simulink model "divider4bit"  (R2020a)
settings: Solver=VariableStepAuto  StartTime=0.0  StopTime=10.0  RelTol=1e-3
libraries: simulink_extras x4
(part 1 of 2)
settings Model: Creator=kishan  LastModifiedBy=kishan

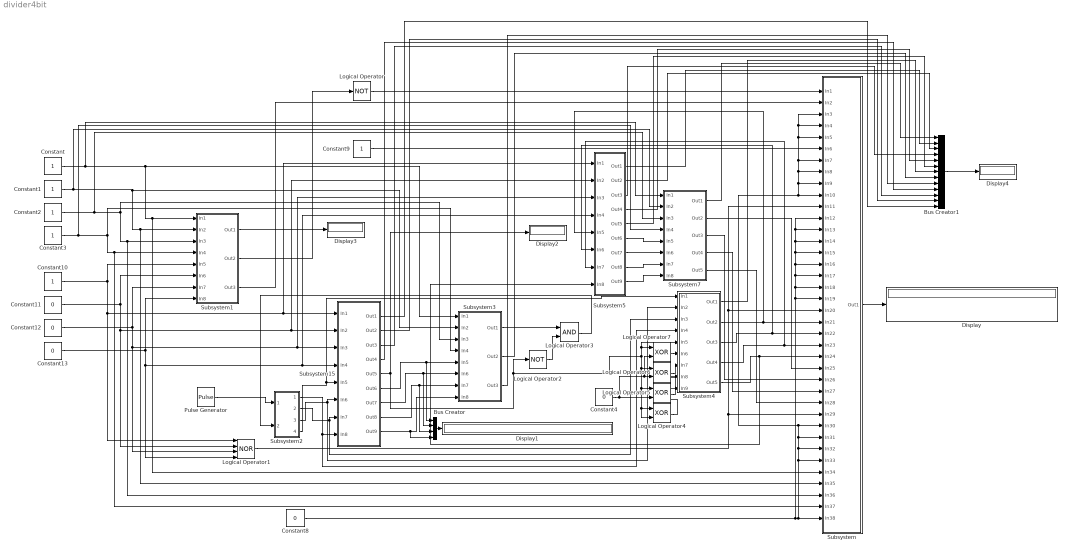
== system divider4bit ==
  Bus Creator : BusCreator  Inputs=4
  Bus Creator1 : BusCreator  Inputs=13
  Constant{,1..3,10} (5 alike) : Constant  OutDataTypeStr=boolean
  Constant11 : Constant  Value=0  OutDataTypeStr=boolean
  Constant12 : Constant  Value=0  OutDataTypeStr=boolean
  Constant13 : Constant  Value=0  OutDataTypeStr=boolean
  Constant4 : Constant  Value=0
  Constant8 : Constant  Value=0
  Constant9 : Constant
  Display{,1..4} (5 alike) : Display
  Logical Operator : Logic  Operator=NOT  AllPortsSameDT=off  OutDataTypeStr=boolean
  Logical Operator1 : Logic  Operator=NOR  Inputs=4  AllPortsSameDT=off  OutDataTypeStr=boolean
  Logical Operator2 : Logic  Operator=NOT  Inputs=4  AllPortsSameDT=off  OutDataTypeStr=boolean
  Logical Operator3 : Logic  AllPortsSameDT=off  OutDataTypeStr=boolean
  Logical Operator{4..7} (4 alike) : Logic  Operator=XOR  AllPortsSameDT=off  OutDataTypeStr=boolean
  Pulse Generator : DiscretePulseGenerator  PulseType=Time based  Period=0.1  PulseWidth=5
  Subsystem : Subsystem
  Subsystem1 : Subsystem
  Subsystem15 : Subsystem
  Subsystem2 : Subsystem
  Subsystem3 : Subsystem
  Subsystem4 : Subsystem
  Subsystem5 : Subsystem
  Subsystem7 : Subsystem
  wires:
  Subsystem/1(Out1) -> Display/1
  Constant3/1 -> Subsystem7/4(In4), Subsystem3/4(In4), Subsystem/37(In37), Subsystem1/4(In4)
  Constant13/1 -> Logical Operator1/4, Subsystem5/4(In4), Subsystem15/4(In4), Subsystem1/8(In8)
  Constant12/1 -> Logical Operator1/3, Subsystem5/3(In3), Subsystem15/3(In3), Subsystem1/7(In7)
  Constant11/1 -> Logical Operator1/2, Subsystem5/2(In2), Subsystem15/2(In2), Subsystem1/6(In6)
  Constant/1 -> Subsystem7/1(In1), Subsystem3/1(In1), Subsystem/34(In34), Subsystem1/1(In1)
  Constant2/1 -> Subsystem7/3(In3), Subsystem3/3(In3), Subsystem/36(In36), Subsystem1/3(In3)
  Subsystem1/3(Out3) -> Subsystem/2(In2)
  Subsystem1/2(Out2) -> Logical Operator/1
  Logical Operator/1 -> Subsystem/1(In1)
  Constant9/1 -> Subsystem/6(In6)
  Logical Operator1/1 -> Subsystem/29(In29), Subsystem/20(In20), Subsystem/11(In11)
  Subsystem15/9(Out9) -> Bus Creator/4, Subsystem3/8(In8)
  Subsystem15/8(Out8) -> Bus Creator/3, Subsystem3/7(In7)
  Subsystem15/7(Out7) -> Bus Creator/2, Subsystem3/6(In6)
  Subsystem15/6(Out6) -> Bus Creator/1, Subsystem3/5(In5)
  Subsystem2/1(Out1) -> Subsystem4/4(In4), Subsystem15/8(In8)
  Subsystem2/2(Out2) -> Subsystem4/3(In3), Subsystem15/7(In7)
  Subsystem2/3(Out3) -> Subsystem4/2(In2), Subsystem15/6(In6)
  Subsystem2/4(Out4) -> Subsystem4/1(In1), Subsystem15/5(In5)
  Pulse Generator/1 -> Subsystem2/1(In1)
  Logical Operator3/1 -> Subsystem2/2(In2)
  Bus Creator/1 -> Display1/1
  Logical Operator2/1 -> Logical Operator3/2
  Subsystem3/1(Out1) -> Logical Operator3/1
  Constant4/1 -> Logical Operator7/2, Logical Operator6/2, Logical Operator5/2
  Logical Operator4/1 -> Subsystem4/9(In9)
  Subsystem4/2(Out2) -> Subsystem5/5(In5), Subsystem/21(In21)
  Subsystem4/3(Out3) -> Subsystem5/6(In6), Subsystem/22(In22)
  Subsystem4/4(Out4) -> Subsystem5/7(In7), Subsystem/23(In23)
  Subsystem4/5(Out5) -> Subsystem/24(In24), Subsystem5/8(In8)
  Subsystem15/5(Out5) -> Logical Operator2/1, Logical Operator5/1, Logical Operator4/2, Logical Operator4/1, Logical Operator6/1, Logical Operator7/1, Subsystem4/5(In5), Display2/1
  Logical Operator5/1 -> Subsystem4/8(In8)
  Logical Operator6/1 -> Subsystem4/7(In7)
  Logical Operator7/1 -> Subsystem4/6(In6)
  Constant10/1 -> Logical Operator1/1, Subsystem5/1(In1), Subsystem15/1(In1), Subsystem1/5(In5)
  Constant1/1 -> Subsystem7/2(In2), Subsystem3/2(In2), Subsystem/35(In35), Subsystem1/2(In2)
  Subsystem5/6(Out6) -> Subsystem7/5(In5)
  Subsystem5/7(Out7) -> Subsystem7/6(In6)
  Subsystem5/8(Out8) -> Subsystem7/7(In7)
  Subsystem5/9(Out9) -> Subsystem7/8(In8)
  Subsystem7/2(Out2) -> Subsystem/25(In25)
  Subsystem7/3(Out3) -> Subsystem/26(In26)
  Subsystem7/4(Out4) -> Subsystem/27(In27)
  Subsystem7/5(Out5) -> Subsystem/28(In28)
  Subsystem1/1(Out1) -> Display3/1
  Constant8/1 -> Subsystem/19(In19), Subsystem/18(In18), Subsystem/17(In17), Subsystem/16(In16), Subsystem/15(In15), Subsystem/14(In14), Subsystem/13(In13), Subsystem/12(In12), Subsystem/38(In38), Subsystem/32(In32), Subsystem/10(In10), Subsystem/9(In9), Subsystem/8(In8), Subsystem/7(In7), Subsystem/5(In5), Subsystem/4(In4), Subsystem/3(In3), Subsystem/30(In30), Subsystem/31(In31), Subsystem/33(In33)
  Bus Creator1/1 -> Display4/1
  Subsystem7/1(Out1) -> Bus Creator1/1
  Subsystem5/1(Out1) -> Bus Creator1/2
  Subsystem5/2(Out2) -> Bus Creator1/3
  Subsystem5/3(Out3) -> Bus Creator1/4
  Subsystem5/4(Out4) -> Bus Creator1/5
  Subsystem5/5(Out5) -> Bus Creator1/6
  Subsystem4/1(Out1) -> Bus Creator1/7
  Subsystem3/2(Out2) -> Bus Creator1/8
  Subsystem3/3(Out3) -> Bus Creator1/9
  Subsystem15/4(Out4) -> Bus Creator1/10
  Subsystem15/3(Out3) -> Bus Creator1/11
  Subsystem15/2(Out2) -> Bus Creator1/12
  Subsystem15/1(Out1) -> Bus Creator1/13

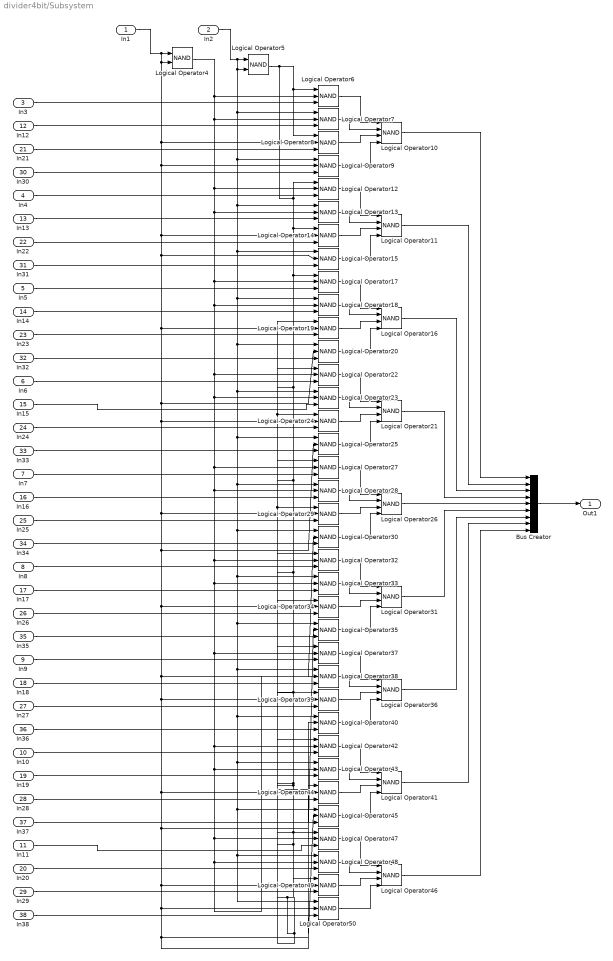
== system divider4bit/Subsystem ==
  In1 : Inport
  In2 : Inport  Port=2
  In3 : Inport  Port=3
  In4 : Inport  Port=4
  In5 : Inport  Port=5
  In6 : Inport  Port=6
  In7 : Inport  Port=7
  In8 : Inport  Port=8
  In9 : Inport  Port=9
  In10 : Inport  Port=10
  In11 : Inport  Port=11
  In12 : Inport  Port=12
  In13 : Inport  Port=13
  In14 : Inport  Port=14
  In15 : Inport  Port=15
  In16 : Inport  Port=16
  In17 : Inport  Port=17
  In18 : Inport  Port=18
  In19 : Inport  Port=19
  In20 : Inport  Port=20
  In21 : Inport  Port=21
  In22 : Inport  Port=22
  In23 : Inport  Port=23
  In24 : Inport  Port=24
  In25 : Inport  Port=25
  In26 : Inport  Port=26
  In27 : Inport  Port=27
  In28 : Inport  Port=28
  In29 : Inport  Port=29
  In30 : Inport  Port=30
  In31 : Inport  Port=31
  In32 : Inport  Port=32
  In33 : Inport  Port=33
  In34 : Inport  Port=34
  In35 : Inport  Port=35
  In36 : Inport  Port=36
  In37 : Inport  Port=37
  In38 : Inport  Port=38
  Bus Creator : BusCreator  Inputs=9
  Logical Operator{10..11,16,21,26,31,36,41,46} (9 alike) : Logic  Operator=NAND  Inputs=4  AllPortsSameDT=off  OutDataTypeStr=boolean
  Logical Operator{6..9,12..15,17..20,22..25,27..30,32..35,37..40,42..45,47..50} (36 alike) : Logic  Operator=NAND  Inputs=3  AllPortsSameDT=off  OutDataTypeStr=boolean
  Logical Operator4 : Logic  Operator=NAND  AllPortsSameDT=off  OutDataTypeStr=boolean
  Logical Operator5 : Logic  Operator=NAND  AllPortsSameDT=off  OutDataTypeStr=boolean
  Out1 : Outport
  wires:
  Logical Operator28/1 -> Logical Operator26/2
  Logical Operator49/1 -> Logical Operator46/3
  In15/1 -> Logical Operator23/3
  In30/1 -> Logical Operator9/3
  Logical Operator33/1 -> Logical Operator31/2
  Logical Operator32/1 -> Logical Operator31/1
  Logical Operator43/1 -> Logical Operator41/2
  Logical Operator37/1 -> Logical Operator36/1
  Logical Operator24/1 -> Logical Operator21/3
  In33/1 -> Logical Operator25/3
  Logical Operator45/1 -> Logical Operator41/4
  Logical Operator42/1 -> Logical Operator41/1
  In37/1 -> Logical Operator45/3
  Logical Operator44/1 -> Logical Operator41/3
  Logical Operator30/1 -> Logical Operator26/4
  In19/1 -> Logical Operator43/3
  In28/1 -> Logical Operator44/3
  Logical Operator34/1 -> Logical Operator31/3
  In38/1 -> Logical Operator50/3
  Logical Operator11/1 -> Bus Creator/2
  Logical Operator22/1 -> Logical Operator21/1
  In18/1 -> Logical Operator38/3
  In22/1 -> Logical Operator14/3
  In14/1 -> Logical Operator18/3
  Logical Operator19/1 -> Logical Operator16/3
  In32/1 -> Logical Operator20/3
  Logical Operator20/1 -> Logical Operator16/4
  Logical Operator48/1 -> Logical Operator46/2
  Logical Operator13/1 -> Logical Operator11/2
  Logical Operator25/1 -> Logical Operator21/4
  In24/1 -> Logical Operator24/3
  In25/1 -> Logical Operator29/3
  In7/1 -> Logical Operator27/3
  In21/1 -> Logical Operator8/3
  Logical Operator23/1 -> Logical Operator21/2
  In8/1 -> Logical Operator32/3
  Logical Operator17/1 -> Logical Operator16/1
  In29/1 -> Logical Operator49/3
  Logical Operator36/1 -> Bus Creator/7
  Logical Operator16/1 -> Bus Creator/3
  In26/1 -> Logical Operator34/3
  Logical Operator50/1 -> Logical Operator46/4
  In17/1 -> Logical Operator33/3
  In3/1 -> Logical Operator6/3
  In4/1 -> Logical Operator12/3
  Logical Operator14/1 -> Logical Operator11/3
  Logical Operator46/1 -> Bus Creator/9
  Logical Operator9/1 -> Logical Operator10/4
  In5/1 -> Logical Operator17/3
  Bus Creator/1 -> Out1/1
  Logical Operator35/1 -> Logical Operator31/4
  Logical Operator26/1 -> Bus Creator/5
  Logical Operator10/1 -> Bus Creator/1
  Logical Operator40/1 -> Logical Operator36/4
  In36/1 -> Logical Operator40/3
  Logical Operator39/1 -> Logical Operator36/3
  In35/1 -> Logical Operator35/3
  Logical Operator29/1 -> Logical Operator26/3
  In2/1 -> Logical Operator50/1, Logical Operator48/1, Logical Operator45/1, Logical Operator43/1, Logical Operator40/1, Logical Operator38/1, Logical Operator35/1, Logical Operator33/1, Logical Operator30/1, Logical Operator28/1, Logical Operator25/1, Logical Operator23/1, Logical Operator20/1, Logical Operator18/1, Logical Operator15/1, Logical Operator13/1, Logical Operator9/1, Logical Operator7/1, Logical Operator5/2, Logical Operator5/1
  Logical Operator38/1 -> Logical Operator36/2
  Logical Operator18/1 -> Logical Operator16/2
  Logical Operator15/1 -> Logical Operator11/4
  In16/1 -> Logical Operator28/3
  Logical Operator27/1 -> Logical Operator26/1
  In27/1 -> Logical Operator39/3
  In20/1 -> Logical Operator48/3
  In10/1 -> Logical Operator42/3
  Logical Operator47/1 -> Logical Operator46/1
  Logical Operator31/1 -> Bus Creator/6
  Logical Operator41/1 -> Bus Creator/8
  In31/1 -> Logical Operator15/3
  Logical Operator8/1 -> Logical Operator10/3
  Logical Operator6/1 -> Logical Operator10/1
  In34/1 -> Logical Operator30/3
  Logical Operator12/1 -> Logical Operator11/1
  In11/1 -> Logical Operator47/3
  In13/1 -> Logical Operator13/3
  Logical Operator7/1 -> Logical Operator10/2
  In12/1 -> Logical Operator7/3
  In23/1 -> Logical Operator19/3
  Logical Operator4/1 -> Logical Operator38/2, Logical Operator48/2, Logical Operator47/2, Logical Operator43/2, Logical Operator42/2, Logical Operator37/2, Logical Operator33/2, Logical Operator32/2, Logical Operator28/2, Logical Operator27/2, Logical Operator23/2, Logical Operator22/2, Logical Operator18/2, Logical Operator17/2, Logical Operator13/2, Logical Operator12/2, Logical Operator7/2, Logical Operator6/2
  Logical Operator21/1 -> Bus Creator/4
  Logical Operator5/1 -> Logical Operator22/1, Logical Operator24/1, Logical Operator29/1, Logical Operator27/1, Logical Operator47/1, Logical Operator49/1, Logical Operator44/1, Logical Operator42/1, Logical Operator37/1, Logical Operator39/1, Logical Operator34/1, Logical Operator32/1, Logical Operator19/1, Logical Operator17/1, Logical Operator14/1, Logical Operator12/1, Logical Operator8/1, Logical Operator6/1
  In9/1 -> Logical Operator37/3
  In1/1 -> Logical Operator40/2, Logical Operator45/2, Logical Operator50/2, Logical Operator49/2, Logical Operator35/2, Logical Operator44/2, Logical Operator39/2, Logical Operator30/2, Logical Operator34/2, Logical Operator25/2, Logical Operator29/2, Logical Operator24/2, Logical Operator20/2, Logical Operator19/2, Logical Operator15/2, Logical Operator14/2, Logical Operator9/2, Logical Operator8/2, Logical Operator4/2, Logical Operator4/1
  In6/1 -> Logical Operator22/3

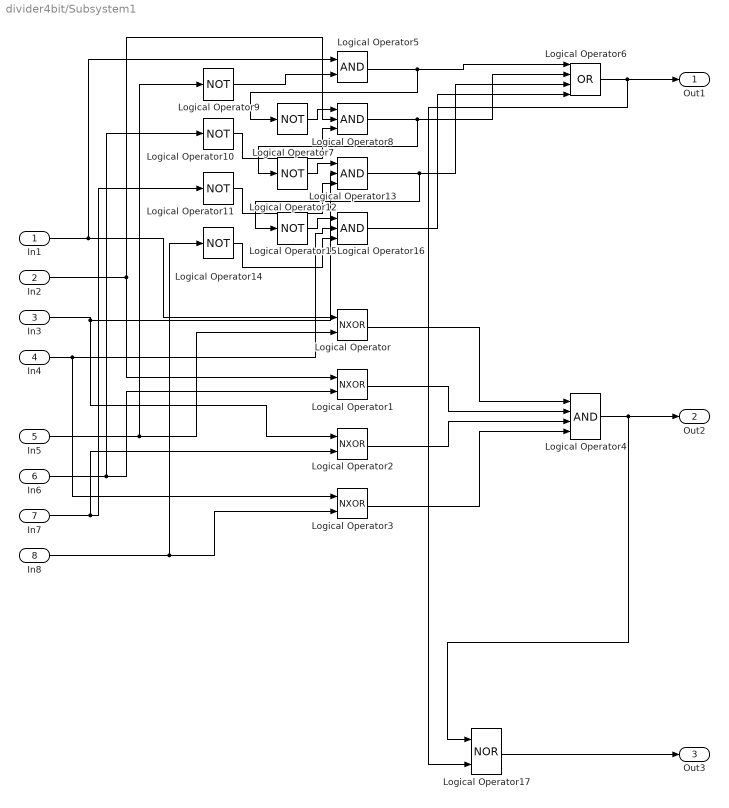
== system divider4bit/Subsystem1 ==
  In1 : Inport
  In2 : Inport  Port=2
  In3 : Inport  Port=3
  In4 : Inport  Port=4
  In5 : Inport  Port=5
  In6 : Inport  Port=6
  In7 : Inport  Port=7
  In8 : Inport  Port=8
  Logical Operator{,1..3} (4 alike) : Logic  Operator=NXOR  AllPortsSameDT=off  OutDataTypeStr=boolean
  Logical Operator{7,9..12,14..15} (7 alike) : Logic  Operator=NOT  Inputs=3  AllPortsSameDT=off  OutDataTypeStr=boolean
  Logical Operator13 : Logic  Inputs=3  AllPortsSameDT=off  OutDataTypeStr=boolean
  Logical Operator16 : Logic  Inputs=3  AllPortsSameDT=off  OutDataTypeStr=boolean
  Logical Operator17 : Logic  Operator=NOR  AllPortsSameDT=off  OutDataTypeStr=boolean
  Logical Operator4 : Logic  Inputs=4  AllPortsSameDT=off  OutDataTypeStr=boolean
  Logical Operator5 : Logic  AllPortsSameDT=off  OutDataTypeStr=boolean
  Logical Operator6 : Logic  Operator=OR  Inputs=4  AllPortsSameDT=off  OutDataTypeStr=boolean
  Logical Operator8 : Logic  Inputs=3  AllPortsSameDT=off  OutDataTypeStr=boolean
  Out1 : Outport
  Out2 : Outport  Port=2
  Out3 : Outport  Port=3
  wires:
  Logical Operator7/1 -> Logical Operator8/1
  Logical Operator17/1 -> Out3/1
  Logical Operator16/1 -> Logical Operator6/4
  Logical Operator12/1 -> Logical Operator13/1
  In7/1 -> Logical Operator11/1, Logical Operator2/2
  Logical Operator4/1 -> Out2/1, Logical Operator17/1
  In1/1 -> Logical Operator5/1, Logical Operator/1
  Logical Operator3/1 -> Logical Operator4/4
  Logical Operator5/1 -> Logical Operator7/1, Logical Operator6/1
  Logical Operator6/1 -> Out1/1, Logical Operator17/2
  In5/1 -> Logical Operator9/1, Logical Operator/2
  In3/1 -> Logical Operator13/2, Logical Operator2/1
  Logical Operator/1 -> Logical Operator4/1
  In6/1 -> Logical Operator10/1, Logical Operator1/2
  Logical Operator1/1 -> Logical Operator4/2
  In4/1 -> Logical Operator16/2, Logical Operator3/1
  In2/1 -> Logical Operator8/2, Logical Operator1/1
  Logical Operator15/1 -> Logical Operator16/1
  In8/1 -> Logical Operator14/1, Logical Operator3/2
  Logical Operator13/1 -> Logical Operator15/1, Logical Operator6/3
  Logical Operator11/1 -> Logical Operator13/3
  Logical Operator8/1 -> Logical Operator12/1, Logical Operator6/2
  Logical Operator2/1 -> Logical Operator4/3
  Logical Operator9/1 -> Logical Operator5/2
  Logical Operator14/1 -> Logical Operator16/3
  Logical Operator10/1 -> Logical Operator8/3

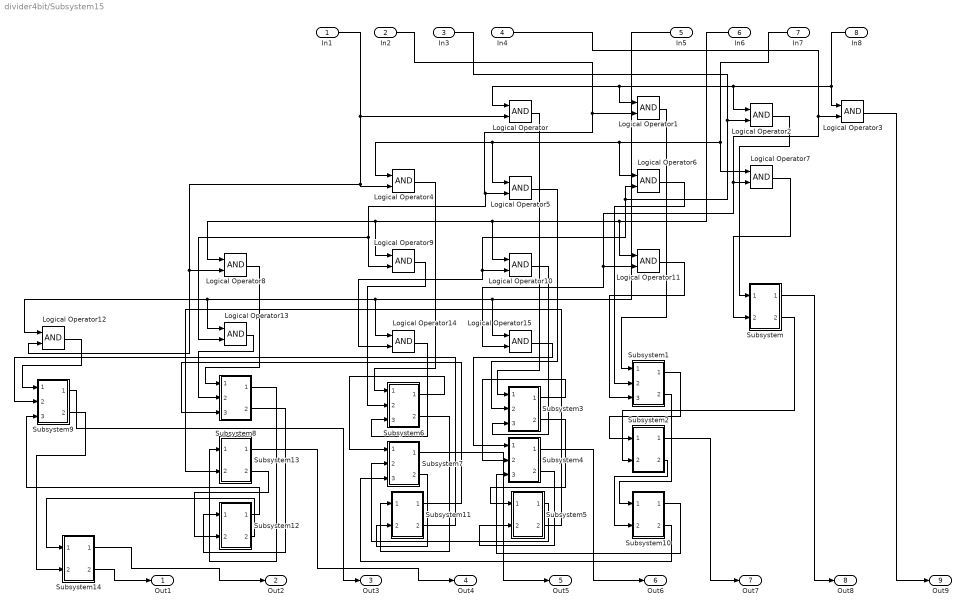
== system divider4bit/Subsystem15 ==
  In1 : Inport
  In2 : Inport  Port=2
  In3 : Inport  Port=3
  In4 : Inport  Port=4
  In5 : Inport  Port=5
  In6 : Inport  Port=6
  In7 : Inport  Port=7
  In8 : Inport  Port=8
  Logical Operator{,1..15} (16 alike) : Logic  AllPortsSameDT=off  OutDataTypeStr=boolean
  Subsystem : Subsystem
  Subsystem1 : Subsystem
  Subsystem10 : Subsystem
  Subsystem11 : Subsystem
  Subsystem12 : Subsystem
  Subsystem13 : Subsystem
  Subsystem14 : Subsystem
  Subsystem2 : Subsystem
  Subsystem3 : Subsystem
  Subsystem4 : Subsystem
  Subsystem5 : Subsystem
  Subsystem6 : Subsystem
  Subsystem7 : Subsystem
  Subsystem8 : Subsystem
  Subsystem9 : Subsystem
  Out1 : Outport
  Out2 : Outport  Port=2
  Out3 : Outport  Port=3
  Out4 : Outport  Port=4
  Out5 : Outport  Port=5
  Out6 : Outport  Port=6
  Out7 : Outport  Port=7
  Out8 : Outport  Port=8
  Out9 : Outport  Port=9
  wires:
  Subsystem11/2(Out2) -> Subsystem9/2(In2)
  Logical Operator7/1 -> Subsystem/2(In2)
  Subsystem4/2(Out2) -> Subsystem5/2(In2)
  Logical Operator13/1 -> Subsystem8/2(In2)
  Subsystem12/1(Out1) -> Subsystem9/3(In3)
  Logical Operator/1 -> Subsystem3/1(In1)
  Subsystem3/1(Out1) -> Subsystem4/2(In2)
  Subsystem14/1(Out1) -> Out2/1
  Logical Operator4/1 -> Subsystem6/1(In1)
  Subsystem1/2(Out2) -> Subsystem10/1(In1)
  Subsystem5/1(Out1) -> Subsystem7/2(In2)
  Subsystem10/2(Out2) -> Subsystem7/3(In3)
  In3/1 -> Logical Operator6/2, Logical Operator14/2, Logical Operator10/2, Logical Operator2/2
  Subsystem8/2(Out2) -> Subsystem12/1(In1)
  Subsystem4/1(Out1) -> Out6/1
  Logical Operator6/1 -> Subsystem1/2(In2)
  Subsystem13/1(Out1) -> Out4/1
  Subsystem2/1(Out1) -> Out7/1
  Subsystem/1(Out1) -> Out8/1
  In5/1 -> Logical Operator12/1, Logical Operator13/1, Logical Operator14/1, Logical Operator15/1
  In1/1 -> Logical Operator12/2, Logical Operator8/2, Logical Operator4/2, Logical Operator/2
  Logical Operator2/1 -> Subsystem/1(In1)
  Subsystem/2(Out2) -> Subsystem2/2(In2)
  Logical Operator3/1 -> Out9/1
  In2/1 -> Logical Operator9/2, Logical Operator13/2, Logical Operator5/2, Logical Operator1/2
  In6/1 -> Logical Operator8/1, Logical Operator9/1, Logical Operator10/1, Logical Operator11/1
  In8/1 -> Logical Operator/1, Logical Operator1/1, Logical Operator2/1, Logical Operator3/1
  Subsystem13/2(Out2) -> Subsystem12/2(In2)
  Logical Operator1/1 -> Subsystem1/1(In1)
  In7/1 -> Logical Operator4/1, Logical Operator5/1, Logical Operator6/1, Logical Operator7/1
  Logical Operator11/1 -> Subsystem1/3(In3)
  Subsystem12/2(Out2) -> Subsystem14/1(In1)
  Logical Operator12/1 -> Subsystem9/1(In1)
  Subsystem10/1(Out1) -> Subsystem4/3(In3)
  Logical Operator15/1 -> Subsystem4/1(In1)
  Logical Operator5/1 -> Subsystem3/2(In2)
  Subsystem7/1(Out1) -> Out5/1
  Subsystem6/2(Out2) -> Subsystem11/1(In1)
  Logical Operator8/1 -> Subsystem8/1(In1)
  Subsystem3/2(Out2) -> Subsystem5/1(In1)
  In4/1 -> Logical Operator15/2, Logical Operator11/2, Logical Operator7/2, Logical Operator3/2
  Subsystem9/1(Out1) -> Out3/1
  Logical Operator14/1 -> Subsystem6/3(In3)
  Subsystem9/2(Out2) -> Subsystem14/2(In2)
  Subsystem11/1(Out1) -> Subsystem8/3(In3)
  Subsystem8/1(Out1) -> Subsystem13/1(In1)
  Subsystem1/1(Out1) -> Subsystem2/1(In1)
  Subsystem2/2(Out2) -> Subsystem10/2(In2)
  Subsystem6/1(Out1) -> Subsystem7/1(In1)
  Subsystem5/2(Out2) -> Subsystem13/2(In2)
  Subsystem14/2(Out2) -> Out1/1
  Logical Operator10/1 -> Subsystem3/3(In3)
  Logical Operator9/1 -> Subsystem6/2(In2)
  Subsystem7/2(Out2) -> Subsystem11/2(In2)

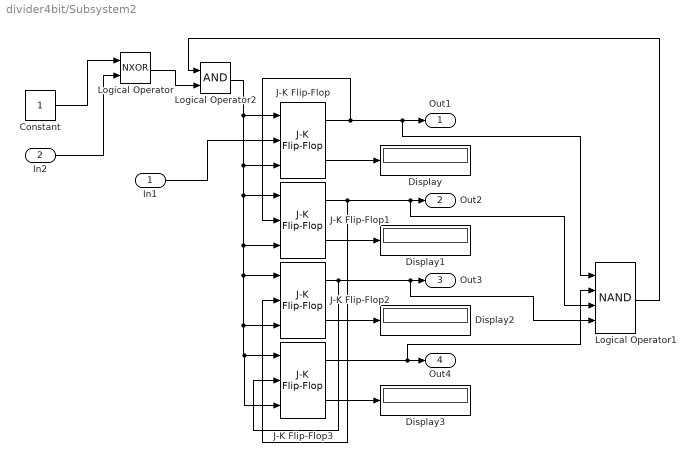
== system divider4bit/Subsystem2 ==
  In1 : Inport
  In2 : Inport  Port=2
  Constant : Constant  OutDataTypeStr=boolean
  Display{,1..3} (4 alike) : Display
  J-K Flip-Flop{,1..3} (4 alike) : simulink_extras/Flip Flops/J-K Flip-Flop  initial_condition=0
  Logical Operator : Logic  Operator=NXOR  AllPortsSameDT=off  OutDataTypeStr=boolean
  Logical Operator1 : Logic  Operator=NAND  Inputs=4  AllPortsSameDT=off  OutDataTypeStr=boolean
  Logical Operator2 : Logic  AllPortsSameDT=off  OutDataTypeStr=boolean
  Out1 : Outport
  Out2 : Outport  Port=2
  Out3 : Outport  Port=3
  Out4 : Outport  Port=4
  wires:
  J-K Flip-Flop1/2 -> Display1/1
  J-K Flip-Flop3/2 -> Display3/1
  J-K Flip-Flop2/2 -> Display2/1
  J-K Flip-Flop3/1 -> Logical Operator1/2, Out4/1
  J-K Flip-Flop/2 -> Display/1
  J-K Flip-Flop1/1 -> J-K Flip-Flop2/2, Logical Operator1/3, Out2/1
  J-K Flip-Flop2/1 -> J-K Flip-Flop3/2, Logical Operator1/4, Out3/1
  In1/1 -> J-K Flip-Flop/2
  J-K Flip-Flop/1 -> J-K Flip-Flop1/2, Logical Operator1/1, Out1/1
  Logical Operator2/1 -> J-K Flip-Flop3/3, J-K Flip-Flop3/1, J-K Flip-Flop2/3, J-K Flip-Flop2/1, J-K Flip-Flop1/3, J-K Flip-Flop1/1, J-K Flip-Flop/3, J-K Flip-Flop/1
  Constant/1 -> Logical Operator/1
  In2/1 -> Logical Operator/2
  Logical Operator/1 -> Logical Operator2/2
  Logical Operator1/1 -> Logical Operator2/1

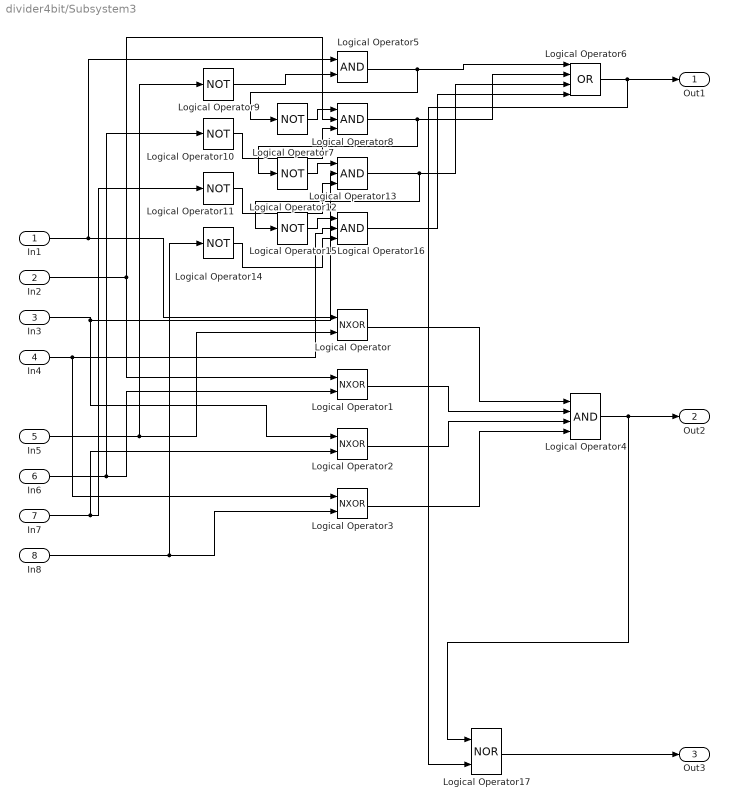
== system divider4bit/Subsystem3 ==
  In1 : Inport
  In2 : Inport  Port=2
  In3 : Inport  Port=3
  In4 : Inport  Port=4
  In5 : Inport  Port=5
  In6 : Inport  Port=6
  In7 : Inport  Port=7
  In8 : Inport  Port=8
  Logical Operator{,1..3} (4 alike) : Logic  Operator=NXOR  AllPortsSameDT=off  OutDataTypeStr=boolean
  Logical Operator{7,9..12,14..15} (7 alike) : Logic  Operator=NOT  Inputs=3  AllPortsSameDT=off  OutDataTypeStr=boolean
  Logical Operator13 : Logic  Inputs=3  AllPortsSameDT=off  OutDataTypeStr=boolean
  Logical Operator16 : Logic  Inputs=3  AllPortsSameDT=off  OutDataTypeStr=boolean
  Logical Operator17 : Logic  Operator=NOR  AllPortsSameDT=off  OutDataTypeStr=boolean
  Logical Operator4 : Logic  Inputs=4  AllPortsSameDT=off  OutDataTypeStr=boolean
  Logical Operator5 : Logic  AllPortsSameDT=off  OutDataTypeStr=boolean
  Logical Operator6 : Logic  Operator=OR  Inputs=4  AllPortsSameDT=off  OutDataTypeStr=boolean
  Logical Operator8 : Logic  Inputs=3  AllPortsSameDT=off  OutDataTypeStr=boolean
  Out1 : Outport
  Out2 : Outport  Port=2
  Out3 : Outport  Port=3
  wires:
  Logical Operator7/1 -> Logical Operator8/1
  Logical Operator17/1 -> Out3/1
  Logical Operator16/1 -> Logical Operator6/4
  Logical Operator12/1 -> Logical Operator13/1
  In7/1 -> Logical Operator11/1, Logical Operator2/2
  Logical Operator4/1 -> Out2/1, Logical Operator17/1
  In1/1 -> Logical Operator5/1, Logical Operator/1
  Logical Operator3/1 -> Logical Operator4/4
  Logical Operator5/1 -> Logical Operator7/1, Logical Operator6/1
  Logical Operator6/1 -> Out1/1, Logical Operator17/2
  In5/1 -> Logical Operator9/1, Logical Operator/2
  In3/1 -> Logical Operator13/2, Logical Operator2/1
  Logical Operator/1 -> Logical Operator4/1
  In6/1 -> Logical Operator10/1, Logical Operator1/2
  Logical Operator1/1 -> Logical Operator4/2
  In4/1 -> Logical Operator16/2, Logical Operator3/1
  In2/1 -> Logical Operator8/2, Logical Operator1/1
  Logical Operator15/1 -> Logical Operator16/1
  In8/1 -> Logical Operator14/1, Logical Operator3/2
  Logical Operator13/1 -> Logical Operator15/1, Logical Operator6/3
  Logical Operator11/1 -> Logical Operator13/3
  Logical Operator8/1 -> Logical Operator12/1, Logical Operator6/2
  Logical Operator2/1 -> Logical Operator4/3
  Logical Operator9/1 -> Logical Operator5/2
  Logical Operator14/1 -> Logical Operator16/3
  Logical Operator10/1 -> Logical Operator8/3

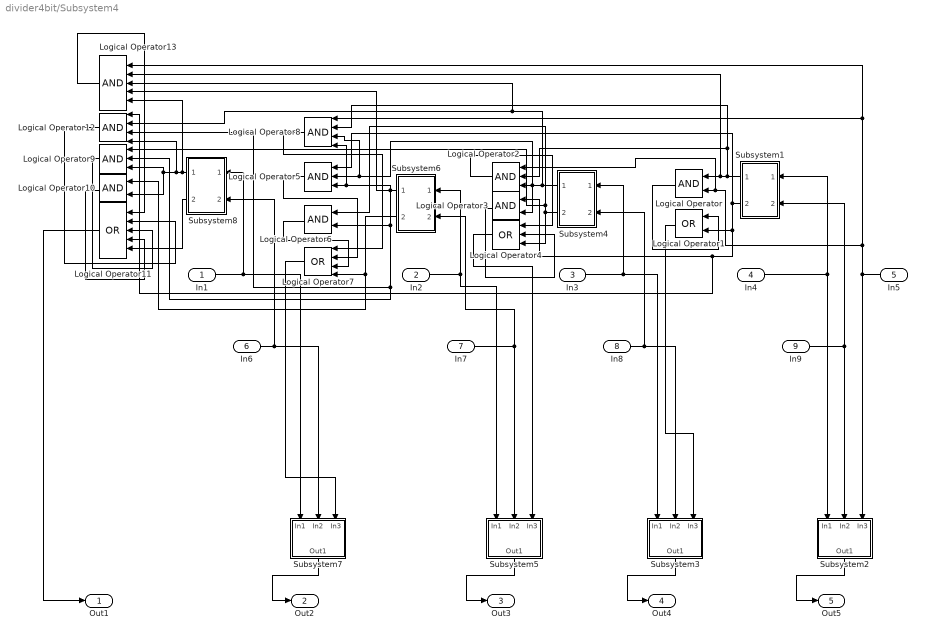
== system divider4bit/Subsystem4 ==
  In1 : Inport
  In2 : Inport  Port=2
  In3 : Inport  Port=3
  In4 : Inport  Port=4
  In5 : Inport  Port=5
  In6 : Inport  Port=6
  In7 : Inport  Port=7
  In8 : Inport  Port=8
  In9 : Inport  Port=9
  Logical Operator{,3,6,10} (4 alike) : Logic  AllPortsSameDT=off  OutDataTypeStr=boolean
  Logical Operator1 : Logic  Operator=OR  AllPortsSameDT=off  OutDataTypeStr=boolean
  Logical Operator11 : Logic  Operator=OR  Inputs=5  AllPortsSameDT=off  OutDataTypeStr=boolean
  Logical Operator12 : Logic  Inputs=4  AllPortsSameDT=off  OutDataTypeStr=boolean
  Logical Operator13 : Logic  Inputs=5  AllPortsSameDT=off  OutDataTypeStr=boolean
  Logical Operator2 : Logic  Inputs=3  AllPortsSameDT=off  OutDataTypeStr=boolean
  Logical Operator4 : Logic  Operator=OR  Inputs=3  AllPortsSameDT=off  OutDataTypeStr=boolean
  Logical Operator5 : Logic  Inputs=3  AllPortsSameDT=off  OutDataTypeStr=boolean
  Logical Operator7 : Logic  Operator=OR  Inputs=4  AllPortsSameDT=off  OutDataTypeStr=boolean
  Logical Operator8 : Logic  Inputs=4  AllPortsSameDT=off  OutDataTypeStr=boolean
  Logical Operator9 : Logic  Inputs=3  AllPortsSameDT=off  OutDataTypeStr=boolean
  Subsystem1 : Subsystem
  Subsystem2 : Subsystem
  Subsystem3 : Subsystem
  Subsystem4 : Subsystem
  Subsystem5 : Subsystem
  Subsystem6 : Subsystem
  Subsystem7 : Subsystem
  Subsystem8 : Subsystem
  Out1 : Outport
  Out2 : Outport  Port=2
  Out3 : Outport  Port=3
  Out4 : Outport  Port=4
  Out5 : Outport  Port=5
  wires:
  Logical Operator11/1 -> Out1/1
  Logical Operator5/1 -> Logical Operator7/2
  Subsystem5/1(Out1) -> Out3/1
  Logical Operator9/1 -> Logical Operator11/3
  Logical Operator/1 -> Logical Operator1/1
  In6/1 -> Subsystem7/2(In2), Subsystem8/2(In2)
  Logical Operator6/1 -> Logical Operator7/3
  In3/1 -> Subsystem3/1(In1), Subsystem4/1(In1)
  In9/1 -> Subsystem2/2(In2), Subsystem1/2(In2)
  Subsystem6/2(Out2) -> Logical Operator10/1, Logical Operator7/4
  Subsystem8/2(Out2) -> Logical Operator11/5
  Logical Operator7/1 -> Subsystem7/3(In3)
  In8/1 -> Subsystem3/2(In2), Subsystem4/2(In2)
  Subsystem1/1(Out1) -> Logical Operator8/2, Logical Operator2/2, Logical Operator13/2, Logical Operator/1
  In1/1 -> Subsystem8/1(In1), Subsystem7/1(In1)
  Logical Operator4/1 -> Subsystem5/3(In3)
  Subsystem4/2(Out2) -> Logical Operator9/1, Logical Operator6/1, Logical Operator4/3
  Subsystem4/1(Out1) -> Logical Operator8/3, Logical Operator5/2, Logical Operator3/2, Logical Operator2/3, Logical Operator13/3, Logical Operator12/2
  In2/1 -> Subsystem6/1(In1), Subsystem5/1(In1)
  In7/1 -> Subsystem5/2(In2), Subsystem6/2(In2)
  In5/1 -> Subsystem2/3(In3), Logical Operator13/1, Logical Operator8/1, Logical Operator2/1, Logical Operator/2
  Subsystem7/1(Out1) -> Out2/1
  Logical Operator3/1 -> Logical Operator4/2
  Subsystem2/1(Out1) -> Out5/1
  Logical Operator8/1 -> Logical Operator7/1
  In4/1 -> Subsystem2/1(In1), Subsystem1/1(In1)
  Logical Operator13/1 -> Logical Operator11/1
  Logical Operator12/1 -> Logical Operator11/2
  Subsystem3/1(Out1) -> Out4/1
  Subsystem8/1(Out1) -> Logical Operator13/5, Logical Operator12/4, Logical Operator10/2, Logical Operator9/3
  Logical Operator2/1 -> Logical Operator4/1
  Logical Operator1/1 -> Subsystem3/3(In3)
  Logical Operator10/1 -> Logical Operator11/4
  Subsystem1/2(Out2) -> Logical Operator12/1, Logical Operator3/1, Logical Operator1/2, Logical Operator5/1
  Subsystem6/1(Out1) -> Logical Operator13/4, Logical Operator12/3, Logical Operator9/2, Logical Operator6/2, Logical Operator8/4, Logical Operator5/3

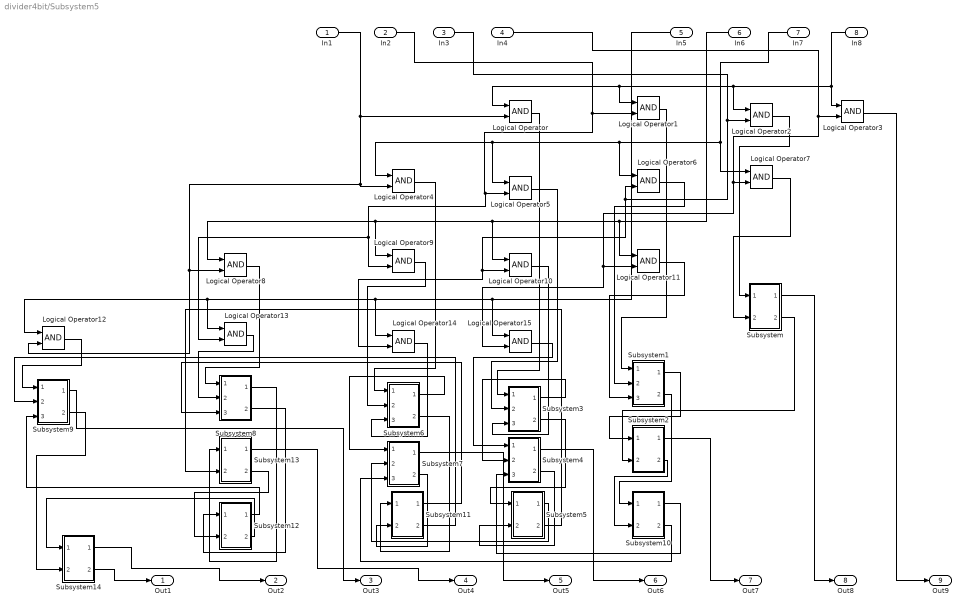
== system divider4bit/Subsystem5 ==
  In1 : Inport
  In2 : Inport  Port=2
  In3 : Inport  Port=3
  In4 : Inport  Port=4
  In5 : Inport  Port=5
  In6 : Inport  Port=6
  In7 : Inport  Port=7
  In8 : Inport  Port=8
  Logical Operator{,1..15} (16 alike) : Logic  AllPortsSameDT=off  OutDataTypeStr=boolean
  Subsystem : Subsystem
  Subsystem1 : Subsystem
  Subsystem10 : Subsystem
  Subsystem11 : Subsystem
  Subsystem12 : Subsystem
  Subsystem13 : Subsystem
  Subsystem14 : Subsystem
  Subsystem2 : Subsystem
  Subsystem3 : Subsystem
  Subsystem4 : Subsystem
  Subsystem5 : Subsystem
  Subsystem6 : Subsystem
  Subsystem7 : Subsystem
  Subsystem8 : Subsystem
  Subsystem9 : Subsystem
  Out1 : Outport
  Out2 : Outport  Port=2
  Out3 : Outport  Port=3
  Out4 : Outport  Port=4
  Out5 : Outport  Port=5
  Out6 : Outport  Port=6
  Out7 : Outport  Port=7
  Out8 : Outport  Port=8
  Out9 : Outport  Port=9
  wires:
  Subsystem11/2(Out2) -> Subsystem9/2(In2)
  Logical Operator7/1 -> Subsystem/2(In2)
  Subsystem4/2(Out2) -> Subsystem5/2(In2)
  Logical Operator13/1 -> Subsystem8/2(In2)
  Subsystem12/1(Out1) -> Subsystem9/3(In3)
  Logical Operator/1 -> Subsystem3/1(In1)
  Subsystem3/1(Out1) -> Subsystem4/2(In2)
  Subsystem14/1(Out1) -> Out2/1
  Logical Operator4/1 -> Subsystem6/1(In1)
  Subsystem1/2(Out2) -> Subsystem10/1(In1)
  Subsystem5/1(Out1) -> Subsystem7/2(In2)
  Subsystem10/2(Out2) -> Subsystem7/3(In3)
  In3/1 -> Logical Operator6/2, Logical Operator14/2, Logical Operator10/2, Logical Operator2/2
  Subsystem8/2(Out2) -> Subsystem12/1(In1)
  Subsystem4/1(Out1) -> Out6/1
  Logical Operator6/1 -> Subsystem1/2(In2)
  Subsystem13/1(Out1) -> Out4/1
  Subsystem2/1(Out1) -> Out7/1
  Subsystem/1(Out1) -> Out8/1
  In5/1 -> Logical Operator12/1, Logical Operator13/1, Logical Operator14/1, Logical Operator15/1
  In1/1 -> Logical Operator12/2, Logical Operator8/2, Logical Operator4/2, Logical Operator/2
  Logical Operator2/1 -> Subsystem/1(In1)
  Subsystem/2(Out2) -> Subsystem2/2(In2)
  Logical Operator3/1 -> Out9/1
  In2/1 -> Logical Operator9/2, Logical Operator13/2, Logical Operator5/2, Logical Operator1/2
  In6/1 -> Logical Operator8/1, Logical Operator9/1, Logical Operator10/1, Logical Operator11/1
  In8/1 -> Logical Operator/1, Logical Operator1/1, Logical Operator2/1, Logical Operator3/1
  Subsystem13/2(Out2) -> Subsystem12/2(In2)
  Logical Operator1/1 -> Subsystem1/1(In1)
  In7/1 -> Logical Operator4/1, Logical Operator5/1, Logical Operator6/1, Logical Operator7/1
  Logical Operator11/1 -> Subsystem1/3(In3)
  Subsystem12/2(Out2) -> Subsystem14/1(In1)
  Logical Operator12/1 -> Subsystem9/1(In1)
  Subsystem10/1(Out1) -> Subsystem4/3(In3)
  Logical Operator15/1 -> Subsystem4/1(In1)
  Logical Operator5/1 -> Subsystem3/2(In2)
  Subsystem7/1(Out1) -> Out5/1
  Subsystem6/2(Out2) -> Subsystem11/1(In1)
  Logical Operator8/1 -> Subsystem8/1(In1)
  Subsystem3/2(Out2) -> Subsystem5/1(In1)
  In4/1 -> Logical Operator15/2, Logical Operator11/2, Logical Operator7/2, Logical Operator3/2
  Subsystem9/1(Out1) -> Out3/1
  Logical Operator14/1 -> Subsystem6/3(In3)
  Subsystem9/2(Out2) -> Subsystem14/2(In2)
  Subsystem11/1(Out1) -> Subsystem8/3(In3)
  Subsystem8/1(Out1) -> Subsystem13/1(In1)
  Subsystem1/1(Out1) -> Subsystem2/1(In1)
  Subsystem2/2(Out2) -> Subsystem10/2(In2)
  Subsystem6/1(Out1) -> Subsystem7/1(In1)
  Subsystem5/2(Out2) -> Subsystem13/2(In2)
  Subsystem14/2(Out2) -> Out1/1
  Logical Operator10/1 -> Subsystem3/3(In3)
  Logical Operator9/1 -> Subsystem6/2(In2)
  Subsystem7/2(Out2) -> Subsystem11/2(In2)

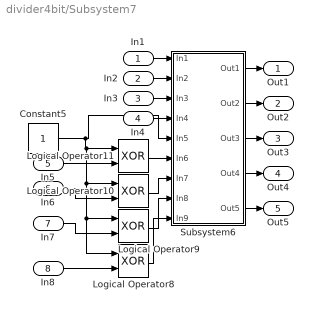
== system divider4bit/Subsystem7 ==
  In1 : Inport
  In2 : Inport  Port=2
  In3 : Inport  Port=3
  In4 : Inport  Port=4
  In5 : Inport  Port=5
  In6 : Inport  Port=6
  In7 : Inport  Port=7
  In8 : Inport  Port=8
  Constant5 : Constant
  Logical Operator{8..11} (4 alike) : Logic  Operator=XOR  AllPortsSameDT=off  OutDataTypeStr=boolean
  Subsystem6 : Subsystem
  Out1 : Outport
  Out2 : Outport  Port=2
  Out3 : Outport  Port=3
  Out4 : Outport  Port=4
  Out5 : Outport  Port=5
  wires:
  Subsystem6/4(Out4) -> Out4/1
  Logical Operator11/1 -> Subsystem6/6(In6)
  Logical Operator9/1 -> Subsystem6/8(In8)
  In6/1 -> Logical Operator10/2
  In8/1 -> Logical Operator8/2
  Subsystem6/1(Out1) -> Out1/1
  Logical Operator10/1 -> Subsystem6/7(In7)
  Subsystem6/3(Out3) -> Out3/1
  Constant5/1 -> Logical Operator8/1, Logical Operator9/1, Logical Operator10/1, Logical Operator11/1, Subsystem6/5(In5)
  In1/1 -> Subsystem6/1(In1)
  Logical Operator8/1 -> Subsystem6/9(In9)
  Subsystem6/5(Out5) -> Out5/1
  In7/1 -> Logical Operator9/2
  In3/1 -> Subsystem6/3(In3)
  In2/1 -> Subsystem6/2(In2)
  Subsystem6/2(Out2) -> Out2/1
  In4/1 -> Subsystem6/4(In4)
  In5/1 -> Logical Operator11/2

== system divider4bit/Subsystem15/Subsystem ==
  In1 : Inport
  In2 : Inport  Port=2
  Logical Operator1 : Logic  Operator=XOR  AllPortsSameDT=off  OutDataTypeStr=boolean
  Logical Operator2 : Logic  AllPortsSameDT=off  OutDataTypeStr=boolean
  Out1 : Outport
  Out2 : Outport  Port=2
  wires:
  In1/1 -> Logical Operator2/1, Logical Operator1/1
  Logical Operator1/1 -> Out1/1
  Logical Operator2/1 -> Out2/1
  In2/1 -> Logical Operator1/2, Logical Operator2/2

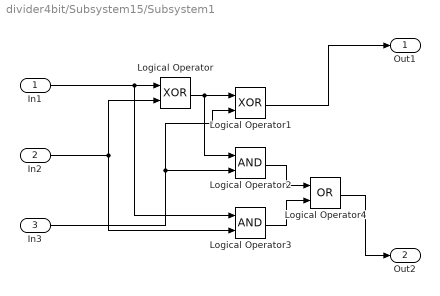
== system divider4bit/Subsystem15/Subsystem1 ==
  In1 : Inport
  In2 : Inport  Port=2
  In3 : Inport  Port=3
  Logical Operator : Logic  Operator=XOR  AllPortsSameDT=off  OutDataTypeStr=boolean
  Logical Operator1 : Logic  Operator=XOR  AllPortsSameDT=off  OutDataTypeStr=boolean
  Logical Operator2 : Logic  AllPortsSameDT=off  OutDataTypeStr=boolean
  Logical Operator3 : Logic  AllPortsSameDT=off  OutDataTypeStr=boolean
  Logical Operator4 : Logic  Operator=OR  AllPortsSameDT=off  OutDataTypeStr=boolean
  Out1 : Outport
  Out2 : Outport  Port=2
  wires:
  Logical Operator1/1 -> Out1/1
  Logical Operator2/1 -> Logical Operator4/1
  Logical Operator4/1 -> Out2/1
  In3/1 -> Logical Operator2/2, Logical Operator1/2
  In2/1 -> Logical Operator3/2, Logical Operator/2
  In1/1 -> Logical Operator3/1, Logical Operator/1
  Logical Operator3/1 -> Logical Operator4/2
  Logical Operator/1 -> Logical Operator2/1, Logical Operator1/1

== system divider4bit/Subsystem15/Subsystem10 ==
  In1 : Inport
  In2 : Inport  Port=2
  Logical Operator1 : Logic  Operator=XOR  AllPortsSameDT=off  OutDataTypeStr=boolean
  Logical Operator2 : Logic  AllPortsSameDT=off  OutDataTypeStr=boolean
  Out1 : Outport
  Out2 : Outport  Port=2
  wires:
  In1/1 -> Logical Operator2/1, Logical Operator1/1
  Logical Operator1/1 -> Out1/1
  Logical Operator2/1 -> Out2/1
  In2/1 -> Logical Operator1/2, Logical Operator2/2

== system divider4bit/Subsystem15/Subsystem11 ==
  In1 : Inport
  In2 : Inport  Port=2
  Logical Operator1 : Logic  Operator=XOR  AllPortsSameDT=off  OutDataTypeStr=boolean
  Logical Operator2 : Logic  AllPortsSameDT=off  OutDataTypeStr=boolean
  Out1 : Outport
  Out2 : Outport  Port=2
  wires:
  In1/1 -> Logical Operator2/1, Logical Operator1/1
  Logical Operator1/1 -> Out1/1
  Logical Operator2/1 -> Out2/1
  In2/1 -> Logical Operator1/2, Logical Operator2/2

== system divider4bit/Subsystem15/Subsystem12 ==
  In1 : Inport
  In2 : Inport  Port=2
  Logical Operator1 : Logic  Operator=XOR  AllPortsSameDT=off  OutDataTypeStr=boolean
  Logical Operator2 : Logic  AllPortsSameDT=off  OutDataTypeStr=boolean
  Out1 : Outport
  Out2 : Outport  Port=2
  wires:
  In1/1 -> Logical Operator2/1, Logical Operator1/1
  Logical Operator1/1 -> Out1/1
  Logical Operator2/1 -> Out2/1
  In2/1 -> Logical Operator1/2, Logical Operator2/2

== system divider4bit/Subsystem15/Subsystem13 ==
  In1 : Inport
  In2 : Inport  Port=2
  Logical Operator1 : Logic  Operator=XOR  AllPortsSameDT=off  OutDataTypeStr=boolean
  Logical Operator2 : Logic  AllPortsSameDT=off  OutDataTypeStr=boolean
  Out1 : Outport
  Out2 : Outport  Port=2
  wires:
  In1/1 -> Logical Operator2/1, Logical Operator1/1
  Logical Operator1/1 -> Out1/1
  Logical Operator2/1 -> Out2/1
  In2/1 -> Logical Operator1/2, Logical Operator2/2

== system divider4bit/Subsystem15/Subsystem14 ==
  In1 : Inport
  In2 : Inport  Port=2
  Logical Operator1 : Logic  Operator=XOR  AllPortsSameDT=off  OutDataTypeStr=boolean
  Logical Operator2 : Logic  AllPortsSameDT=off  OutDataTypeStr=boolean
  Out1 : Outport
  Out2 : Outport  Port=2
  wires:
  In1/1 -> Logical Operator2/1, Logical Operator1/1
  Logical Operator1/1 -> Out1/1
  Logical Operator2/1 -> Out2/1
  In2/1 -> Logical Operator1/2, Logical Operator2/2

== system divider4bit/Subsystem15/Subsystem2 ==
  In1 : Inport
  In2 : Inport  Port=2
  Logical Operator1 : Logic  Operator=XOR  AllPortsSameDT=off  OutDataTypeStr=boolean
  Logical Operator2 : Logic  AllPortsSameDT=off  OutDataTypeStr=boolean
  Out1 : Outport
  Out2 : Outport  Port=2
  wires:
  In1/1 -> Logical Operator2/1, Logical Operator1/1
  Logical Operator1/1 -> Out1/1
  Logical Operator2/1 -> Out2/1
  In2/1 -> Logical Operator1/2, Logical Operator2/2

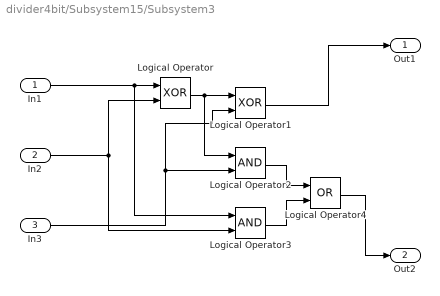
== system divider4bit/Subsystem15/Subsystem3 ==
  In1 : Inport
  In2 : Inport  Port=2
  In3 : Inport  Port=3
  Logical Operator : Logic  Operator=XOR  AllPortsSameDT=off  OutDataTypeStr=boolean
  Logical Operator1 : Logic  Operator=XOR  AllPortsSameDT=off  OutDataTypeStr=boolean
  Logical Operator2 : Logic  AllPortsSameDT=off  OutDataTypeStr=boolean
  Logical Operator3 : Logic  AllPortsSameDT=off  OutDataTypeStr=boolean
  Logical Operator4 : Logic  Operator=OR  AllPortsSameDT=off  OutDataTypeStr=boolean
  Out1 : Outport
  Out2 : Outport  Port=2
  wires:
  Logical Operator1/1 -> Out1/1
  Logical Operator2/1 -> Logical Operator4/1
  Logical Operator4/1 -> Out2/1
  In3/1 -> Logical Operator2/2, Logical Operator1/2
  In2/1 -> Logical Operator3/2, Logical Operator/2
  In1/1 -> Logical Operator3/1, Logical Operator/1
  Logical Operator3/1 -> Logical Operator4/2
  Logical Operator/1 -> Logical Operator2/1, Logical Operator1/1

== system divider4bit/Subsystem15/Subsystem4 ==
  In1 : Inport
  In2 : Inport  Port=2
  In3 : Inport  Port=3
  Logical Operator : Logic  Operator=XOR  AllPortsSameDT=off  OutDataTypeStr=boolean
  Logical Operator1 : Logic  Operator=XOR  AllPortsSameDT=off  OutDataTypeStr=boolean
  Logical Operator2 : Logic  AllPortsSameDT=off  OutDataTypeStr=boolean
  Logical Operator3 : Logic  AllPortsSameDT=off  OutDataTypeStr=boolean
  Logical Operator4 : Logic  Operator=OR  AllPortsSameDT=off  OutDataTypeStr=boolean
  Out1 : Outport
  Out2 : Outport  Port=2
  wires:
  Logical Operator1/1 -> Out1/1
  Logical Operator2/1 -> Logical Operator4/1
  Logical Operator4/1 -> Out2/1
  In3/1 -> Logical Operator2/2, Logical Operator1/2
  In2/1 -> Logical Operator3/2, Logical Operator/2
  In1/1 -> Logical Operator3/1, Logical Operator/1
  Logical Operator3/1 -> Logical Operator4/2
  Logical Operator/1 -> Logical Operator2/1, Logical Operator1/1

== system divider4bit/Subsystem15/Subsystem5 ==
  In1 : Inport
  In2 : Inport  Port=2
  Logical Operator1 : Logic  Operator=XOR  AllPortsSameDT=off  OutDataTypeStr=boolean
  Logical Operator2 : Logic  AllPortsSameDT=off  OutDataTypeStr=boolean
  Out1 : Outport
  Out2 : Outport  Port=2
  wires:
  In1/1 -> Logical Operator2/1, Logical Operator1/1
  Logical Operator1/1 -> Out1/1
  Logical Operator2/1 -> Out2/1
  In2/1 -> Logical Operator1/2, Logical Operator2/2

== system divider4bit/Subsystem15/Subsystem6 ==
  In1 : Inport
  In2 : Inport  Port=2
  In3 : Inport  Port=3
  Logical Operator : Logic  Operator=XOR  AllPortsSameDT=off  OutDataTypeStr=boolean
  Logical Operator1 : Logic  Operator=XOR  AllPortsSameDT=off  OutDataTypeStr=boolean
  Logical Operator2 : Logic  AllPortsSameDT=off  OutDataTypeStr=boolean
  Logical Operator3 : Logic  AllPortsSameDT=off  OutDataTypeStr=boolean
  Logical Operator4 : Logic  Operator=OR  AllPortsSameDT=off  OutDataTypeStr=boolean
  Out1 : Outport
  Out2 : Outport  Port=2
  wires:
  Logical Operator1/1 -> Out1/1
  Logical Operator2/1 -> Logical Operator4/1
  Logical Operator4/1 -> Out2/1
  In3/1 -> Logical Operator2/2, Logical Operator1/2
  In2/1 -> Logical Operator3/2, Logical Operator/2
  In1/1 -> Logical Operator3/1, Logical Operator/1
  Logical Operator3/1 -> Logical Operator4/2
  Logical Operator/1 -> Logical Operator2/1, Logical Operator1/1

== system divider4bit/Subsystem15/Subsystem7 ==
  In1 : Inport
  In2 : Inport  Port=2
  In3 : Inport  Port=3
  Logical Operator : Logic  Operator=XOR  AllPortsSameDT=off  OutDataTypeStr=boolean
  Logical Operator1 : Logic  Operator=XOR  AllPortsSameDT=off  OutDataTypeStr=boolean
  Logical Operator2 : Logic  AllPortsSameDT=off  OutDataTypeStr=boolean
  Logical Operator3 : Logic  AllPortsSameDT=off  OutDataTypeStr=boolean
  Logical Operator4 : Logic  Operator=OR  AllPortsSameDT=off  OutDataTypeStr=boolean
  Out1 : Outport
  Out2 : Outport  Port=2
  wires:
  Logical Operator1/1 -> Out1/1
  Logical Operator2/1 -> Logical Operator4/1
  Logical Operator4/1 -> Out2/1
  In3/1 -> Logical Operator2/2, Logical Operator1/2
  In2/1 -> Logical Operator3/2, Logical Operator/2
  In1/1 -> Logical Operator3/1, Logical Operator/1
  Logical Operator3/1 -> Logical Operator4/2
  Logical Operator/1 -> Logical Operator2/1, Logical Operator1/1

== system divider4bit/Subsystem15/Subsystem8 ==
  In1 : Inport
  In2 : Inport  Port=2
  In3 : Inport  Port=3
  Logical Operator : Logic  Operator=XOR  AllPortsSameDT=off  OutDataTypeStr=boolean
  Logical Operator1 : Logic  Operator=XOR  AllPortsSameDT=off  OutDataTypeStr=boolean
  Logical Operator2 : Logic  AllPortsSameDT=off  OutDataTypeStr=boolean
  Logical Operator3 : Logic  AllPortsSameDT=off  OutDataTypeStr=boolean
  Logical Operator4 : Logic  Operator=OR  AllPortsSameDT=off  OutDataTypeStr=boolean
  Out1 : Outport
  Out2 : Outport  Port=2
  wires:
  Logical Operator1/1 -> Out1/1
  Logical Operator2/1 -> Logical Operator4/1
  Logical Operator4/1 -> Out2/1
  In3/1 -> Logical Operator2/2, Logical Operator1/2
  In2/1 -> Logical Operator3/2, Logical Operator/2
  In1/1 -> Logical Operator3/1, Logical Operator/1
  Logical Operator3/1 -> Logical Operator4/2
  Logical Operator/1 -> Logical Operator2/1, Logical Operator1/1

== system divider4bit/Subsystem15/Subsystem9 ==
  In1 : Inport
  In2 : Inport  Port=2
  In3 : Inport  Port=3
  Logical Operator : Logic  Operator=XOR  AllPortsSameDT=off  OutDataTypeStr=boolean
  Logical Operator1 : Logic  Operator=XOR  AllPortsSameDT=off  OutDataTypeStr=boolean
  Logical Operator2 : Logic  AllPortsSameDT=off  OutDataTypeStr=boolean
  Logical Operator3 : Logic  AllPortsSameDT=off  OutDataTypeStr=boolean
  Logical Operator4 : Logic  Operator=OR  AllPortsSameDT=off  OutDataTypeStr=boolean
  Out1 : Outport
  Out2 : Outport  Port=2
  wires:
  Logical Operator1/1 -> Out1/1
  Logical Operator2/1 -> Logical Operator4/1
  Logical Operator4/1 -> Out2/1
  In3/1 -> Logical Operator2/2, Logical Operator1/2
  In2/1 -> Logical Operator3/2, Logical Operator/2
  In1/1 -> Logical Operator3/1, Logical Operator/1
  Logical Operator3/1 -> Logical Operator4/2
  Logical Operator/1 -> Logical Operator2/1, Logical Operator1/1

== system divider4bit/Subsystem4/Subsystem1 ==
  In1 : Inport
  In2 : Inport  Port=2
  Logical Operator : Logic  Operator=XOR  AllPortsSameDT=off  OutDataTypeStr=boolean
  Logical Operator1 : Logic  AllPortsSameDT=off  OutDataTypeStr=boolean
  Out1 : Outport
  Out2 : Outport  Port=2
  wires:
  In1/1 -> Logical Operator1/1, Logical Operator/1
  Logical Operator1/1 -> Out2/1
  In2/1 -> Logical Operator1/2, Logical Operator/2
  Logical Operator/1 -> Out1/1

== system divider4bit/Subsystem4/Subsystem2 ==
  In1 : Inport
  In2 : Inport  Port=2
  In3 : Inport  Port=3
  Logical Operator2 : Logic  Operator=XOR  AllPortsSameDT=off  OutDataTypeStr=boolean
  Logical Operator3 : Logic  Operator=XOR  AllPortsSameDT=off  OutDataTypeStr=boolean
  Out1 : Outport
  wires:
  In3/1 -> Logical Operator3/2
  In2/1 -> Logical Operator2/2
  In1/1 -> Logical Operator2/1
  Logical Operator2/1 -> Logical Operator3/1
  Logical Operator3/1 -> Out1/1

== system divider4bit/Subsystem4/Subsystem3 ==
  In1 : Inport
  In2 : Inport  Port=2
  In3 : Inport  Port=3
  Logical Operator2 : Logic  Operator=XOR  AllPortsSameDT=off  OutDataTypeStr=boolean
  Logical Operator3 : Logic  Operator=XOR  AllPortsSameDT=off  OutDataTypeStr=boolean
  Out1 : Outport
  wires:
  In3/1 -> Logical Operator3/2
  In2/1 -> Logical Operator2/2
  In1/1 -> Logical Operator2/1
  Logical Operator2/1 -> Logical Operator3/1
  Logical Operator3/1 -> Out1/1

== system divider4bit/Subsystem4/Subsystem4 ==
  In1 : Inport
  In2 : Inport  Port=2
  Logical Operator : Logic  Operator=XOR  AllPortsSameDT=off  OutDataTypeStr=boolean
  Logical Operator1 : Logic  AllPortsSameDT=off  OutDataTypeStr=boolean
  Out1 : Outport
  Out2 : Outport  Port=2
  wires:
  In1/1 -> Logical Operator1/1, Logical Operator/1
  Logical Operator1/1 -> Out2/1
  In2/1 -> Logical Operator1/2, Logical Operator/2
  Logical Operator/1 -> Out1/1

== system divider4bit/Subsystem4/Subsystem5 ==
  In1 : Inport
  In2 : Inport  Port=2
  In3 : Inport  Port=3
  Logical Operator2 : Logic  Operator=XOR  AllPortsSameDT=off  OutDataTypeStr=boolean
  Logical Operator3 : Logic  Operator=XOR  AllPortsSameDT=off  OutDataTypeStr=boolean
  Out1 : Outport
  wires:
  In3/1 -> Logical Operator3/2
  In2/1 -> Logical Operator2/2
  In1/1 -> Logical Operator2/1
  Logical Operator2/1 -> Logical Operator3/1
  Logical Operator3/1 -> Out1/1

== system divider4bit/Subsystem4/Subsystem6 ==
  In1 : Inport
  In2 : Inport  Port=2
  Logical Operator : Logic  Operator=XOR  AllPortsSameDT=off  OutDataTypeStr=boolean
  Logical Operator1 : Logic  AllPortsSameDT=off  OutDataTypeStr=boolean
  Out1 : Outport
  Out2 : Outport  Port=2
  wires:
  In1/1 -> Logical Operator1/1, Logical Operator/1
  Logical Operator1/1 -> Out2/1
  In2/1 -> Logical Operator1/2, Logical Operator/2
  Logical Operator/1 -> Out1/1

== system divider4bit/Subsystem4/Subsystem7 ==
  In1 : Inport
  In2 : Inport  Port=2
  In3 : Inport  Port=3
  Logical Operator2 : Logic  Operator=XOR  AllPortsSameDT=off  OutDataTypeStr=boolean
  Logical Operator3 : Logic  Operator=XOR  AllPortsSameDT=off  OutDataTypeStr=boolean
  Out1 : Outport
  wires:
  In3/1 -> Logical Operator3/2
  In2/1 -> Logical Operator2/2
  In1/1 -> Logical Operator2/1
  Logical Operator2/1 -> Logical Operator3/1
  Logical Operator3/1 -> Out1/1

== system divider4bit/Subsystem4/Subsystem8 ==
  In1 : Inport
  In2 : Inport  Port=2
  Logical Operator : Logic  Operator=XOR  AllPortsSameDT=off  OutDataTypeStr=boolean
  Logical Operator1 : Logic  AllPortsSameDT=off  OutDataTypeStr=boolean
  Out1 : Outport
  Out2 : Outport  Port=2
  wires:
  In1/1 -> Logical Operator1/1, Logical Operator/1
  Logical Operator1/1 -> Out2/1
  In2/1 -> Logical Operator1/2, Logical Operator/2
  Logical Operator/1 -> Out1/1

== system divider4bit/Subsystem5/Subsystem ==
  In1 : Inport
  In2 : Inport  Port=2
  Logical Operator1 : Logic  Operator=XOR  AllPortsSameDT=off  OutDataTypeStr=boolean
  Logical Operator2 : Logic  AllPortsSameDT=off  OutDataTypeStr=boolean
  Out1 : Outport
  Out2 : Outport  Port=2
  wires:
  In1/1 -> Logical Operator2/1, Logical Operator1/1
  Logical Operator1/1 -> Out1/1
  Logical Operator2/1 -> Out2/1
  In2/1 -> Logical Operator1/2, Logical Operator2/2

== system divider4bit/Subsystem5/Subsystem1 ==
  In1 : Inport
  In2 : Inport  Port=2
  In3 : Inport  Port=3
  Logical Operator : Logic  Operator=XOR  AllPortsSameDT=off  OutDataTypeStr=boolean
  Logical Operator1 : Logic  Operator=XOR  AllPortsSameDT=off  OutDataTypeStr=boolean
  Logical Operator2 : Logic  AllPortsSameDT=off  OutDataTypeStr=boolean
  Logical Operator3 : Logic  AllPortsSameDT=off  OutDataTypeStr=boolean
  Logical Operator4 : Logic  Operator=OR  AllPortsSameDT=off  OutDataTypeStr=boolean
  Out1 : Outport
  Out2 : Outport  Port=2
  wires:
  Logical Operator1/1 -> Out1/1
  Logical Operator2/1 -> Logical Operator4/1
  Logical Operator4/1 -> Out2/1
  In3/1 -> Logical Operator2/2, Logical Operator1/2
  In2/1 -> Logical Operator3/2, Logical Operator/2
  In1/1 -> Logical Operator3/1, Logical Operator/1
  Logical Operator3/1 -> Logical Operator4/2
  Logical Operator/1 -> Logical Operator2/1, Logical Operator1/1

== system divider4bit/Subsystem5/Subsystem10 ==
  In1 : Inport
  In2 : Inport  Port=2
  Logical Operator1 : Logic  Operator=XOR  AllPortsSameDT=off  OutDataTypeStr=boolean
  Logical Operator2 : Logic  AllPortsSameDT=off  OutDataTypeStr=boolean
  Out1 : Outport
  Out2 : Outport  Port=2
  wires:
  In1/1 -> Logical Operator2/1, Logical Operator1/1
  Logical Operator1/1 -> Out1/1
  Logical Operator2/1 -> Out2/1
  In2/1 -> Logical Operator1/2, Logical Operator2/2

== system divider4bit/Subsystem5/Subsystem11 ==
  In1 : Inport
  In2 : Inport  Port=2
  Logical Operator1 : Logic  Operator=XOR  AllPortsSameDT=off  OutDataTypeStr=boolean
  Logical Operator2 : Logic  AllPortsSameDT=off  OutDataTypeStr=boolean
  Out1 : Outport
  Out2 : Outport  Port=2
  wires:
  In1/1 -> Logical Operator2/1, Logical Operator1/1
  Logical Operator1/1 -> Out1/1
  Logical Operator2/1 -> Out2/1
  In2/1 -> Logical Operator1/2, Logical Operator2/2

== system divider4bit/Subsystem5/Subsystem12 ==
  In1 : Inport
  In2 : Inport  Port=2
  Logical Operator1 : Logic  Operator=XOR  AllPortsSameDT=off  OutDataTypeStr=boolean
  Logical Operator2 : Logic  AllPortsSameDT=off  OutDataTypeStr=boolean
  Out1 : Outport
  Out2 : Outport  Port=2
  wires:
  In1/1 -> Logical Operator2/1, Logical Operator1/1
  Logical Operator1/1 -> Out1/1
  Logical Operator2/1 -> Out2/1
  In2/1 -> Logical Operator1/2, Logical Operator2/2

== system divider4bit/Subsystem5/Subsystem13 ==
  In1 : Inport
  In2 : Inport  Port=2
  Logical Operator1 : Logic  Operator=XOR  AllPortsSameDT=off  OutDataTypeStr=boolean
  Logical Operator2 : Logic  AllPortsSameDT=off  OutDataTypeStr=boolean
  Out1 : Outport
  Out2 : Outport  Port=2
  wires:
  In1/1 -> Logical Operator2/1, Logical Operator1/1
  Logical Operator1/1 -> Out1/1
  Logical Operator2/1 -> Out2/1
  In2/1 -> Logical Operator1/2, Logical Operator2/2

== system divider4bit/Subsystem5/Subsystem14 ==
  In1 : Inport
  In2 : Inport  Port=2
  Logical Operator1 : Logic  Operator=XOR  AllPortsSameDT=off  OutDataTypeStr=boolean
  Logical Operator2 : Logic  AllPortsSameDT=off  OutDataTypeStr=boolean
  Out1 : Outport
  Out2 : Outport  Port=2
  wires:
  In1/1 -> Logical Operator2/1, Logical Operator1/1
  Logical Operator1/1 -> Out1/1
  Logical Operator2/1 -> Out2/1
  In2/1 -> Logical Operator1/2, Logical Operator2/2

== system divider4bit/Subsystem5/Subsystem2 ==
  In1 : Inport
  In2 : Inport  Port=2
  Logical Operator1 : Logic  Operator=XOR  AllPortsSameDT=off  OutDataTypeStr=boolean
  Logical Operator2 : Logic  AllPortsSameDT=off  OutDataTypeStr=boolean
  Out1 : Outport
  Out2 : Outport  Port=2
  wires:
  In1/1 -> Logical Operator2/1, Logical Operator1/1
  Logical Operator1/1 -> Out1/1
  Logical Operator2/1 -> Out2/1
  In2/1 -> Logical Operator1/2, Logical Operator2/2

== system divider4bit/Subsystem5/Subsystem3 ==
  In1 : Inport
  In2 : Inport  Port=2
  In3 : Inport  Port=3
  Logical Operator : Logic  Operator=XOR  AllPortsSameDT=off  OutDataTypeStr=boolean
  Logical Operator1 : Logic  Operator=XOR  AllPortsSameDT=off  OutDataTypeStr=boolean
  Logical Operator2 : Logic  AllPortsSameDT=off  OutDataTypeStr=boolean
  Logical Operator3 : Logic  AllPortsSameDT=off  OutDataTypeStr=boolean
  Logical Operator4 : Logic  Operator=OR  AllPortsSameDT=off  OutDataTypeStr=boolean
  Out1 : Outport
  Out2 : Outport  Port=2
  wires:
  Logical Operator1/1 -> Out1/1
  Logical Operator2/1 -> Logical Operator4/1
  Logical Operator4/1 -> Out2/1
  In3/1 -> Logical Operator2/2, Logical Operator1/2
  In2/1 -> Logical Operator3/2, Logical Operator/2
  In1/1 -> Logical Operator3/1, Logical Operator/1
  Logical Operator3/1 -> Logical Operator4/2
  Logical Operator/1 -> Logical Operator2/1, Logical Operator1/1
